simulink model "Fans_ClgDem"  (R2016b)
settings: configuration reference "CodeGenConfigSet" (kept outside this file)
values from neighbouring files (symbols this model uses):
  Fans_facVelCor_CUR = Calibration.Parameter    [init_Fans_ClgDem.m]    (also in init_Fans_ClgDem_SIL.m = Simulink.Parameter)
  Fans_facVelCor_CURX = Calibration.Parameter    [init_Fans_ClgDem.m]    (also in init_Fans_ClgDem_SIL.m = Simulink.Parameter)
  Fans_facVelCorErr_C = Calibration.Parameter    [init_Fans_ClgDem.m]    (also in init_Fans_ClgDem_SIL.m = Simulink.Parameter)
  Fans_RmpSlpNeg_C = Calibration.Parameter    [init_Fans_ClgDem.m]    (also in init_Fans_ClgDem_SIL.m = Simulink.Parameter)
  Fans_RmpSlpPos_C = Calibration.Parameter    [init_Fans_ClgDem.m]    (also in init_Fans_ClgDem_SIL.m = Simulink.Parameter)
undefined symbols (not defined in the file or in its folder): FanCtl_nSpdDes2_MAP_CURX, Fans_ClgDem_DT
libraries: CXLib x3
settings Model: Creator=xinchangran  LastModifiedBy=xinchangran
settings ConfigSetRef: SourceLocation=Base Workspace

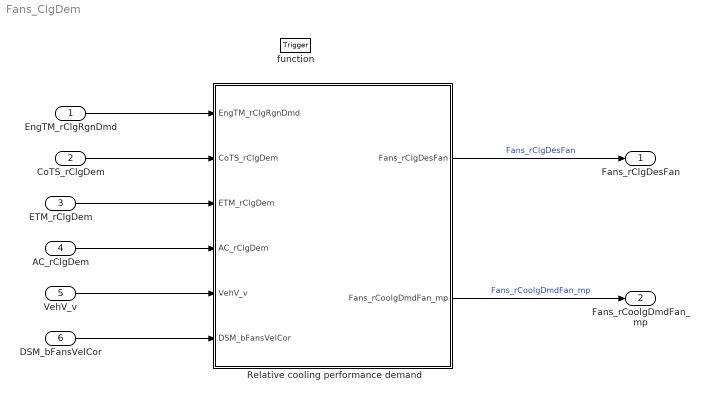
== system Fans_ClgDem ==
  EngTM_rClgRgnDmd : Inport  Tag=%  Description=Cooling demand required to cool the DPF  OutMin=-300  OutMax=300  OutDataTypeStr=Prc_100_rate
  CoTS_rClgDem : Inport  Tag=%  Description=cool demand percent  Port=2  OutMin=-300  OutMax=300  OutDataTypeStr=Prc_100_rate
  ETM_rClgDem : Inport  Tag=%  Description=Relative fan cooling power required by engine cooling  Port=3  OutMin=-300  OutMax=300  OutDataTypeStr=Prc_100_rate
  AC_rClgDem : Inport  Tag=%  Port=4  OutMin=-300  OutMax=300  OutDataTypeStr=Prc_100_rate
  VehV_v : Inport  Tag=km/h  Description=Vehicle speed  Port=5  OutMin=0  OutMax=250  OutDataTypeStr=VehSpeed_km_h
  DSM_bFansVelCor : Inport  Port=6  OutMin=0  OutMax=1  OutDataTypeStr=Dsm
  function : TriggerPort  TriggerType=function-call  VariantControl=Variant
  Relative cooling performance demand : Subsystem
  Fans_rClgDesFan : Outport  Tag=%  Description=Relative cooling performance demand to fan  OutMin=-300  OutMax=300  OutDataTypeStr=Prc_100_rate
  Fans_rCoolgDmdFan_mp : Outport  Tag=%  Description=corrected fan−demand after maximum choice  Port=2  OutMin=-300  OutMax=300  OutDataTypeStr=Prc_100_rate
  wires:
  Relative cooling performance demand/1(Fans_rClgDesFan) -> Fans_rClgDesFan/1  "Fans_rClgDesFan"
  Relative cooling performance demand/2(Fans_rCoolgDmdFan_mp) -> Fans_rCoolgDmdFan_mp/1  "Fans_rCoolgDmdFan_mp"
  EngTM_rClgRgnDmd/1 -> Relative cooling performance demand/1(EngTM_rClgRgnDmd)
  CoTS_rClgDem/1 -> Relative cooling performance demand/2(CoTS_rClgDem)
  ETM_rClgDem/1 -> Relative cooling performance demand/3(ETM_rClgDem)
  AC_rClgDem/1 -> Relative cooling performance demand/4(AC_rClgDem)
  VehV_v/1 -> Relative cooling performance demand/5(VehV_v)
  DSM_bFansVelCor/1 -> Relative cooling performance demand/6(DSM_bFansVelCor)

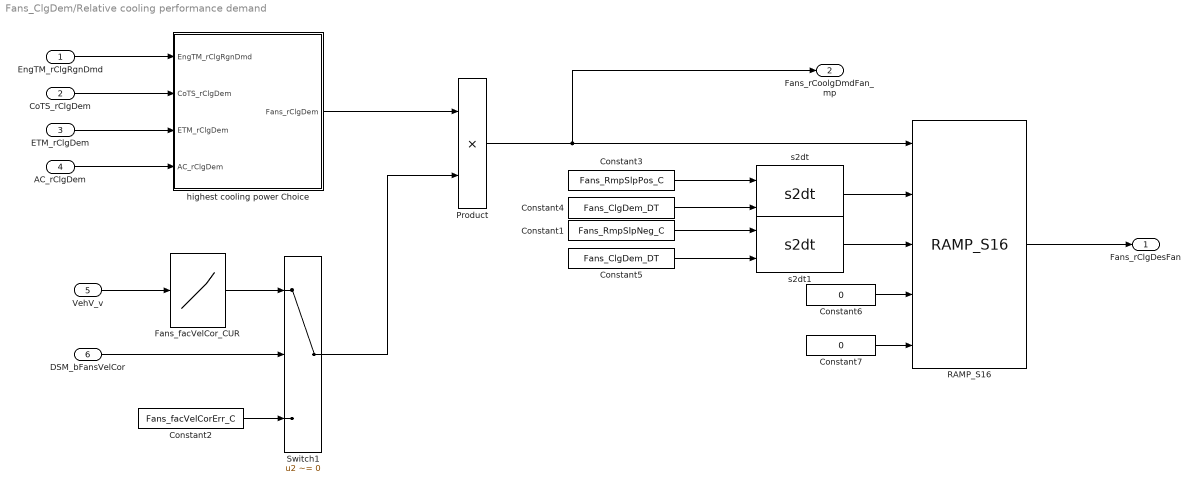
== system Fans_ClgDem/Relative cooling performance demand ==
  EngTM_rClgRgnDmd : Inport
  CoTS_rClgDem : Inport  Port=2
  ETM_rClgDem : Inport  Port=3
  AC_rClgDem : Inport  Port=4
  VehV_v : Inport  Port=5
  DSM_bFansVelCor : Inport  Port=6  OutDataTypeStr=Dsm
  Constant1 : Constant  Value=Fans_RmpSlpNeg_C
  Constant2 : Constant  Value=Fans_facVelCorErr_C
  Constant3 : Constant  Value=Fans_RmpSlpPos_C
  Constant4 : Constant  Value=Fans_ClgDem_DT
  Constant5 : Constant  Value=Fans_ClgDem_DT
  Constant6 : Constant  Value=0  OutDataTypeStr=Inherit: Inherit via back propagation
  Constant7 : Constant  Value=0  OutDataTypeStr=Inherit: Inherit via back propagation
  Fans_facVelCor_CUR : Lookup_n-D  NumberOfTableDimensions=1  BreakpointsForDimension1=Fans_facVelCor_CURX  BreakpointsForDimension2=FanCtl_nSpdDes2_MAP_CURX  BreakpointsForDimension1DataTypeStr=Inherit: Inherit from 'Breakpoint data'  BeginIndexSearchUsingPreviousIndexResult=on  Table=Fans_facVelCor_CUR  ExtrapMethod=Clip  UseLastTableValue=on  InternalRulePriority=Speed  OutDataTypeStr=Inherit: Inherit from 'Table data'  RndMeth=Simplest  SaturateOnIntegerOverflow=on
  Product : Product  OutDataTypeStr=Inherit: Inherit via back propagation  SaturateOnIntegerOverflow=on
  RAMP_S16 : CXLib/RAMP_S16
  Switch1 : Switch  Criteria=u2 ~= 0  SaturateOnIntegerOverflow=on  InputSameDT=on
  highest cooling power Choice : Subsystem
  s2dt : CXLib/s2dt
  s2dt1 : CXLib/s2dt
  Fans_rClgDesFan : Outport
  Fans_rCoolgDmdFan_mp : Outport  Port=2
  wires:
  RAMP_S16/1 -> Fans_rClgDesFan/1
  EngTM_rClgRgnDmd/1 -> highest cooling power Choice/1(EngTM_rClgRgnDmd)
  CoTS_rClgDem/1 -> highest cooling power Choice/2(CoTS_rClgDem)
  ETM_rClgDem/1 -> highest cooling power Choice/3(ETM_rClgDem)
  AC_rClgDem/1 -> highest cooling power Choice/4(AC_rClgDem)
  VehV_v/1 -> Fans_facVelCor_CUR/1
  Fans_facVelCor_CUR/1 -> Switch1/1
  DSM_bFansVelCor/1 -> Switch1/2
  Switch1/1 -> Product/2
  Constant2/1 -> Switch1/3
  s2dt/1 -> RAMP_S16/2
  s2dt1/1 -> RAMP_S16/3
  Constant3/1 -> s2dt/1
  Constant1/1 -> s2dt1/1
  Constant5/1 -> s2dt1/2
  Constant4/1 -> s2dt/2
  Constant7/1 -> RAMP_S16/5
  Constant6/1 -> RAMP_S16/4
  highest cooling power Choice/1(Fans_rClgDem) -> Product/1
  Product/1 -> RAMP_S16/1, Fans_rCoolgDmdFan_mp/1

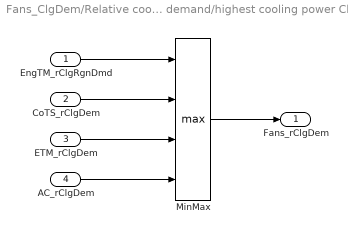
== system Fans_ClgDem/Relative cooling performance demand/highest cooling power Choice ==
  EngTM_rClgRgnDmd : Inport
  CoTS_rClgDem : Inport  Port=2
  ETM_rClgDem : Inport  Port=3
  AC_rClgDem : Inport  Port=4
  MinMax : MinMax  Function=max  Inputs=4
  Fans_rClgDem : Outport
  wires:
  ETM_rClgDem/1 -> MinMax/3
  AC_rClgDem/1 -> MinMax/4
  CoTS_rClgDem/1 -> MinMax/2
  EngTM_rClgRgnDmd/1 -> MinMax/1
  MinMax/1 -> Fans_rClgDem/1
